simulink model "uav_simulation_tarot_r2022a"  (R2022a)
settings: Solver=ode45  StartTime=0.0  StopTime=sim_params.max_sim_time  FixedStep=uav.dynamics_srate  MaxStep=uav.dynamics_srate  MinStep=.001  RelTol=.01
undefined symbols (not defined in the file): deg, DiscIntNeverNeededParam, P_failure, processes, rad, s, sim_params, uav
libraries: aerolibconvert2 x2, shared6dof x1, dspstat3 x1
(part 1 of 2)
settings Model: Creator=Researcher  LastModifiedBy=oem
settings SolverCC: MaxConsecutiveMinStep=10  AlgebraicLoopSolver=TrustRegion
settings DataIOCC: ReturnWorkspaceOutputs=off
settings DebuggingCC: UnconnectedInputMsg=warning  UnconnectedOutputMsg=warning  UnconnectedLineMsg=warning  SFMachineParentedDataDiag=warning  ArithmeticOperatorsInVariantConditions=warning
settings SFSimCC: SimUseLocalCustomCode=off  CustomCodeUndefinedFunction=UseInterfaceOnly
settings RTWCC: RTWUseLocalCustomCode=off

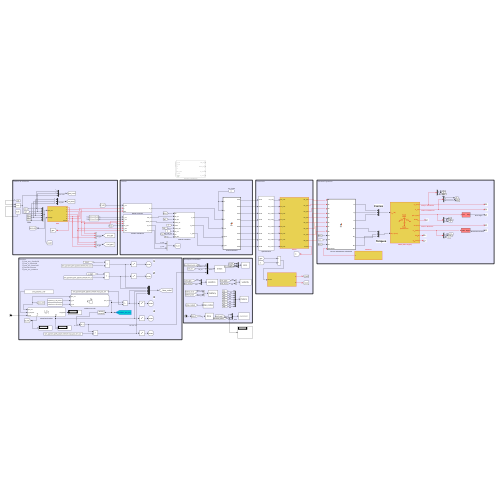
[thumbnail: Simulink's stored preview of the top-level diagram]
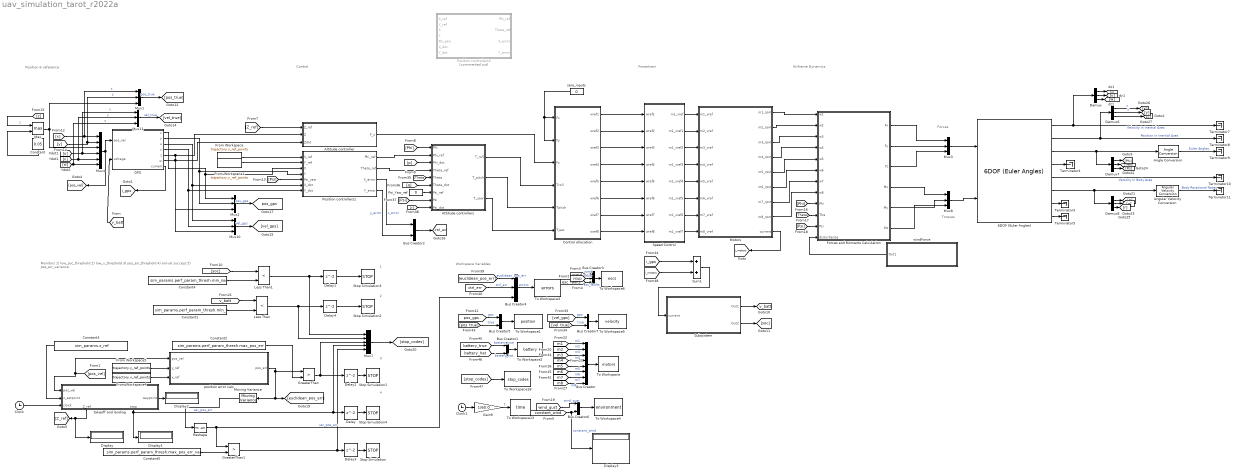
== system uav_simulation_tarot_r2022a ==
  note: Airframe Dynamics
  note: 1
  note: Monitors
      | 	1) low_soc_threshold
      | 	2) low_v_threshold
      | 	3) pos_err_threshold
      | 	4) arrival success
      |       5) pos_err_variance
  note: Powertrain
  note: Control
  note: 2
  note: 3
  note: 4
  note: Position & reference
  note: Workspace Variables
  note: Torques
  note: Forces
  6DOF (Euler Angles) : shared6dof/6DOF (Euler Angles)  units=Metric (MKS)  mtype=Fixed  rep=Quaternion  xme_0=[sim_params.initial_conditions.X, sim_params.initial_conditions.Y, sim_params.initial_conditions.Z]  Vm_0=[0 0 0]  eul_0=[0 0 0]  pm_0=[0 0 0]  mass_0=uav.mass  mass_e=0.5  mass_f=2.0  inertia=uav.airframe.Jb  inertia_e=eye(3)  inertia_f=2*eye(3)  k_quat=1.0  vre_flag=on  abi_flag=off  aMode=0  xme_statename=''  Vm_statename=''  eul_statename=''  quat_statename=''  pm_statename=''  mass_statename=''
      settings: SourceProductBaseCode=AE,PW,DR,MT,VE
  Altitude controller : Subsystem
  Angle Conversion : aerolibconvert2/Angle Conversion  IU=rad  OU=deg
  Angular Velocity Conversion : aerolibconvert2/Angular Velocity Conversion  IU=rad/s  OU=deg/s
  Attitude controllers : Subsystem
  Bus Creator : BusCreator  Inputs=8
  Bus Creator{1..2,5..7} (5 alike) : BusCreator  Inputs=2
  Bus Creator3 : BusCreator  Inputs=3
  Bus Creator4 : BusCreator  Inputs=3
  Clock : Clock
  Clock1 : Clock
  Constant : Constant  Value=0.05
  Constant1 : Constant  Value=sim_params.perf_param_thresh.min_v
  Constant2 : Constant  Value=sim_params.perf_param_thresh.max_pos_err
  Constant3 : Constant  Value=sim_params.z_ref
  Constant4 : Constant  Value=sim_params.perf_param_thresh.min_soc
  Constant5 : Constant  Value=sim_params.perf_param_thresh.max_pos_err_var
  Control allocation : MATLAB Function  TreatAsAtomicUnit=on
  Delay{,1..4} (5 alike) : Delay
  Demux{,6..8} (4 alike) : Demux  Outputs=3
  Display{,1..3} (4 alike) : Display
  Forces and Moments Calculation : MATLAB Function  TreatAsAtomicUnit=on
  From Workspace : FromWorkspace  VariableName=trajectory.x_ref_points
  From Workspace1 : FromWorkspace  VariableName=trajectory.y_ref_points
  From Workspace4 : FromWorkspace  VariableName=trajectory.x_ref_points
  From Workspace5 : FromWorkspace  VariableName=trajectory.y_ref_points
  GPS : Subsystem
  Gain9 : Gain  Gain=1/60.0
  GreaterThan : RelationalOperator  Operator=>  OutDataTypeStr=boolean  RndMeth=Simplest  InputSameDT=off
  GreaterThan1 : RelationalOperator  Operator=>  OutDataTypeStr=boolean  RndMeth=Simplest  InputSameDT=off
  Less Than : RelationalOperator  Operator=<  OutDataTypeStr=boolean  RndMeth=Simplest  InputSameDT=off
  Less Than1 : RelationalOperator  Operator=<  OutDataTypeStr=boolean  RndMeth=Simplest  InputSameDT=off
  Max : MinMax  Function=max  Inputs=2
  Motors : Subsystem
  Moving Variance : dspstat3/Moving Variance  Method=Sliding window  ForgettingFactorPort=off  SpecifyWindowLength=on  WindowLength=250  ForgettingFactor=0.9  SimulateUsing=Code generation
      settings: SourceProductBaseCode=DS
  Mux{1..3,8,10..11} (6 alike) : Mux  Inputs=3
  Mux4 : Mux  Inputs=6
  Mux7 : Mux  Inputs=5
  Position controllers1 : Subsystem
  Position controllers2 : Subsystem  Commented=on
  Psi_Yaw_ref : Constant  Value=0
  Reshape : Reshape
  Speed Control : Subsystem
  Stop Simulation{,1..4} (5 alike) : Stop
  Subsystem : Subsystem
  Sum1 : Sum
  Terminator{3..5,7..11} (8 alike) : Terminator
  To Workspace : ToWorkspace  VariableName=motors  SaveFormat=Timeseries  SampleTime=-1
  To Workspace1 : ToWorkspace  VariableName=position  SaveFormat=Timeseries  SampleTime=-1
  To Workspace13 : ToWorkspace  VariableName=time  SaveFormat=Timeseries  SampleTime=-1
  To Workspace18 : ToWorkspace  VariableName=stop_codes  SaveFormat=Timeseries  SampleTime=-1
  To Workspace2 : ToWorkspace  VariableName=battery  SaveFormat=Timeseries  SampleTime=-1
  To Workspace3 : ToWorkspace  VariableName=errors  SaveFormat=Timeseries  SampleTime=-1
  To Workspace4 : ToWorkspace  VariableName=environment  SaveFormat=Timeseries  SampleTime=-1
  To Workspace5 : ToWorkspace  VariableName=velocity  SaveFormat=Timeseries  SampleTime=-1
  To Workspace6 : ToWorkspace  VariableName=escs  SaveFormat=Timeseries  SampleTime=-1
  position error calc : Stateflow chart  TreatAsAtomicUnit=on
      settings: PortSchema="{\"entries\":[{\"content\":{\"sides\":[{\"content\":{\"connectorIds\":[\"In1\",\"In3\",\"In2\"]},\"type\":\"ConnectorPlacement.EquallySpacedRectSide\",\"uuid\":\"15dd5aaf-db5f-4100-8d44-c6b196b99d7e\"},{\"content\":{\"connectorIds\":[\"Out1\"],\"side\":\"RIGHT\"},\"type\":\"ConnectorPlacement.EquallySpacedRectSide\",\"uuid\":\"60222e26-82e5-4320-be9d-a2c6fe091c2c\"},{\"content\":{\"connectorIds\":[],\"side\":\"TOP\"},\"type\":\"ConnectorPlacement.EquallySpacedRectSide\",\"uuid\":\"f68d0c6c-3e4f-4411-aa05-b15e83a97581\"},{\"content\":{\"connectorIds\":[],\"side\":\"BOTTOM\"},\"type\":\"ConnectorPlacement.EquallySpacedRectSide\",\"uuid\":\"4c051fdf-ae8c-4c56-a072-e71b38b23a79\"}]},\"type\":\"ConnectorPlacement.EquallySpacedConnector\",\"uuid\":\"476607e2-95ee-46d1-bde8-442c90884603\"}],\"packageUris\":[\"http://schema.mathworks.com/mf0/Connector/R2020b\"],\"version\":\"1.0\"}"
  takeoff and landing : Stateflow chart  TreatAsAtomicUnit=on
      settings: PortSchema="{\"entries\":[{\"content\":{\"sides\":[{\"content\":{\"connectorIds\":[\"In1\",\"In2\",\"In3\"]},\"type\":\"ConnectorPlacement.EquallySpacedRectSide\",\"uuid\":\"11e534f3-7296-40bf-aaf5-6b635a6123b7\"},{\"content\":{\"connectorIds\":[\"Out1\"],\"side\":\"RIGHT\"},\"type\":\"ConnectorPlacement.EquallySpacedRectSide\",\"uuid\":\"0c003671-8499-4bdc-80ec-6f06b7f1861b\"},{\"content\":{\"connectorIds\":[],\"side\":\"TOP\"},\"type\":\"ConnectorPlacement.EquallySpacedRectSide\",\"uuid\":\"dd8fb418-d1e6-4628-bf44-6fc4ef2cf7ad\"},{\"content\":{\"connectorIds\":[\"Out2\",\"Out3\"],\"side\":\"BOTTOM\"},\"type\":\"ConnectorPlacement.EquallySpacedRectSide\",\"uuid\":\"62eca2cb-761d-4ce3-a85c-b402bb41b07d\"}]},\"type\":\"ConnectorPlacement.EquallySpacedConnector\",\"uuid\":\"b3efa352-b8bc-43a3-a44e-514725c3dafc\"}],\"packageUris\":[\"http://schema.mathworks.com/mf0/Connector/R2020b\"],\"version\":\"1.0\"}"
  windForce : Subsystem
  zero_inputs : Constant  Value=0
  tag scope: ctrl_err=global, i_gps=global, i_motors=global, pos_gps=global, v_batt=global
  wires:
  [y] -> Mux4/2, Mux1/2  "y"
  [x] -> Mux1/1, Mux4/1  "x"
  Attitude controllers/1(T_roll) -> Control allocation/4(Troll)
  Position controllers1/1(Phi_ref) -> Attitude controllers/2(Phi_ref)
  [r] -> Attitude controllers/9(Psi_dot)
  Attitude controllers/3(T_yaw) -> Control allocation/6(Tyaw)
  Bus Creator2/1 -> [ctrl_err]
  [Psi] -> Position controllers1/5(Psi_yaw)
  Position controllers1/3(X_error) -> Bus Creator2/1  "x_error"
  Attitude controllers/2(T_pitch) -> Control allocation/5(Tpitch)
  [Theta] -> Attitude controllers/5(Theta)
  Position controllers1/2(Theta_ref) -> Attitude controllers/4(Theta_ref)
  Altitude controller/1(F_z) -> Control allocation/3(Fz)
  [Phi] -> Attitude controllers/1(Phi)
  Position controllers1/4(Y_error) -> Bus Creator2/2  "y_error"
  [Psi] -> Attitude controllers/8(Psi)
  zero_inputs/1 -> Control allocation/1(Fx), Control allocation/2(Fy)
  [q] -> Attitude controllers/6(Theta_dot)
  Psi_Yaw_ref/1 -> Attitude controllers/7(Psi_ref)
  [p] -> Attitude controllers/3(Phi_dot)
  Mux7/1 -> [stop_codes]
  Gain9/1 -> To Workspace13/1  "t"
  Delay1/1 -> Stop Simulation3/1
  Constant4/1 -> Less Than1/2
  Clock1/1 -> Gain9/1
  [soc] -> Less Than1/1
  Less Than1/1 -> Delay1/1, Mux7/1
  [stop_codes] -> To Workspace18/1
  [pos_gps] -> Bus Creator5/1  "gps"
  [battery_true] -> Bus Creator1/1  "battery_true"
  [battery_hat] -> Bus Creator1/2  "battery_hat"
  Motors/9(current) -> [i_motors]
  Subsystem/1(Out1) -> [v_batt]
  Subsystem/2(Out2) -> [soc]
  windForce/1(Out1) -> Forces and Moments Calculation/12(disturbance)
  [m2] -> Bus Creator/2  "m2"
  Mux1/1 -> [pos_true]  "pos_true"
  Constant1/1 -> Less Than/2
  [v_batt] -> Less Than/1
  Delay4/1 -> Stop Simulation2/1
  Less Than/1 -> Mux7/2, Delay4/1
  [m1] -> Bus Creator/1  "m1"
  Bus Creator/1 -> To Workspace/1
  [m3] -> Bus Creator/3  "m3"
  [m4] -> Bus Creator/4  "m4"
  [m5] -> Bus Creator/5  "m5"
  [m6] -> Bus Creator/6  "m6"
  [m7] -> Bus Creator/7  "m7"
  [m8] -> Bus Creator/8  "m8"
  [pos_true] -> Bus Creator5/2  "true"
  Mux2/1 -> [pos_gps]  "pos_gps"
  Bus Creator1/1 -> To Workspace2/1
  [euclidean_pos_err] -> Bus Creator4/1  "euclidean_pos_err"
  [ctrl_err] -> Bus Creator4/2  "ctrl_err"
  Bus Creator4/1 -> To Workspace3/1  "errors"
  Bus Creator5/1 -> To Workspace1/1
  [wind_gust] -> Bus Creator6/1  "wind_gust"
  Bus Creator6/1 -> To Workspace4/1
  Forces and Moments Calculation/3(Fz) -> Mux3/3
  Forces and Moments Calculation/6(Mz) -> Mux8/3
  Angle Conversion/1 -> Terminator9/1  "Euler Angles"
  Mux3/1 -> 6DOF (Euler Angles)/1
  Forces and Moments Calculation/5(My) -> Mux8/2
  Angular Velocity Conversion/1 -> Terminator11/1  "Body Rotational Rates"
  Forces and Moments Calculation/2(Fy) -> Mux3/2
  Demux6/2 -> [y]  "y"
  Mux8/1 -> 6DOF (Euler Angles)/2
  6DOF (Euler Angles)/2 -> Terminator8/1, Demux6/1  "Position in Inertial Axes"
  Demux8/1 -> [p]
  Demux/3 -> [w]
  6DOF (Euler Angles)/8 -> Terminator5/1
  Demux6/1 -> [x]  "x"
  Demux7/2 -> [Theta]
  Forces and Moments Calculation/4(Mx) -> Mux8/1
  6DOF (Euler Angles)/7 -> Terminator3/1
  6DOF (Euler Angles)/6 -> Demux8/1, Angular Velocity Conversion/1
  Demux8/3 -> [r]
  Demux7/1 -> [Phi]
  Demux8/2 -> [q]
  6DOF (Euler Angles)/3 -> Demux7/1, Angle Conversion/1
  6DOF (Euler Angles)/4 -> Terminator4/1
  6DOF (Euler Angles)/1 -> Terminator7/1, Demux/1  "Velocity in Inertial Axes"
  Demux6/3 -> [z]
  Forces and Moments Calculation/1(Fx) -> Mux3/1
  6DOF (Euler Angles)/5 -> Terminator10/1  "Velocity in Body Axes"
  Demux7/3 -> [Psi]
  Demux/2 -> [v]
  Demux/1 -> [u]
  Motors/1(m1_rpm) -> Forces and Moments Calculation/1(w1)
  Motors/2(m2_rpm) -> Forces and Moments Calculation/2(w2)
  Motors/3(m3_rpm) -> Forces and Moments Calculation/3(w3)
  Motors/4(m4_rpm) -> Forces and Moments Calculation/4(w4)
  Motors/5(m5_rpm) -> Forces and Moments Calculation/5(w5)
  Motors/6(m6_rpm) -> Forces and Moments Calculation/6(w6)
  Motors/7(m7_rpm) -> Forces and Moments Calculation/7(w7)
  Motors/8(m8_rpm) -> Forces and Moments Calculation/8(w8)
  [Psi] -> Forces and Moments Calculation/11(Psi)
  [Theta] -> Forces and Moments Calculation/10(The)
  [Phi] -> Forces and Moments Calculation/9(Phi)
  [vel_gps] -> Bus Creator7/1  "gps"
  [vel_true] -> Bus Creator7/2  "true"
  Bus Creator7/1 -> To Workspace5/1
  [v] -> Mux11/2, Mux4/5  "y"
  Mux10/1 -> [vel_gps]  "vel_gps"
  [w] -> Mux11/3, Mux4/6  "z"
  [u] -> Mux11/1, Mux4/4  "x"
  Mux11/1 -> [vel_true]  "vel_true"
  GPS/3(u) -> Mux10/1, Position controllers1/6(X_dot)
  GPS/4(v) -> Mux10/2, Position controllers1/7(Y_dot)
  GPS/2(y) -> Mux2/2, Position controllers1/4(Y)
  GPS/1(x) -> Position controllers1/3(X), Mux2/1
  Mux4/1 -> [pos_vel], GPS/1(pos_vel)
  GPS/5(z) -> Mux2/3, Altitude controller/2(Z)
  GPS/6(w) -> Mux10/3, Altitude controller/3(Zdot)
  [v_batt] -> GPS/2(voltage)
  GPS/7(current) -> [i_gps]
  Sum1/1 -> Subsystem/1(current)
  [i_gps] -> Sum1/1
  [i_motors] -> Sum1/2
  Constant/1 -> Max/2
  [z] -> Max/1  "z"
  Max/1 -> Mux4/3, Mux1/3
  Delay/1 -> Stop Simulation4/1
  [pos_vel] -> position error calc/1(pos_vel), takeoff and landing/1(pos_vel)
  takeoff and landing/2(Z_ref) -> Display/1, [Z_ref]
  [Z_ref] -> Altitude controller/1(Z_ref)
  From Workspace5/1 -> position error calc/3(y_ref)
  From Workspace4/1 -> position error calc/2(x_ref)
  Constant2/1 -> GreaterThan/2
  Delay2/1 -> Stop Simulation1/1
  GreaterThan/1 -> Mux7/3, Delay2/1
  takeoff and landing/3(stop) -> Mux7/4, Delay/1, Display1/1
  Control allocation/1(wref1) -> Speed Control/1(wref1)
  Control allocation/2(wref2) -> Speed Control/2(wref2)
  Control allocation/3(wref3) -> Speed Control/3(wref3)
  Control allocation/4(wref4) -> Speed Control/4(wref4)
  Control allocation/5(wref5) -> Speed Control/5(wref5)
  Control allocation/6(wref6) -> Speed Control/6(wref6)
  Control allocation/7(wref7) -> Speed Control/7(wref7)
  Control allocation/8(wref8) -> Speed Control/8(wref8)
  Speed Control/1(m1_vref) -> Motors/1(m1_vref)
  Speed Control/2(m1_vref1) -> Motors/2(m2_vref)
  Speed Control/3(m1_vref2) -> Motors/3(m3_vref)
  Speed Control/4(m1_vref3) -> Motors/4(m4_vref)
  Speed Control/5(m1_vref4) -> Motors/5(m5_vref)
  Speed Control/6(m1_vref5) -> Motors/6(m6_vref)
  Speed Control/7(m1_vref6) -> Motors/7(m7_vref)
  Speed Control/8(m1_vref7) -> Motors/8(m8_vref)
  Constant3/1 -> takeoff and landing/2(z_setpoint)
  Clock/1 -> takeoff and landing/3(clock)
  From Workspace/1 -> Position controllers1/1(X_ref)
  From Workspace1/1 -> Position controllers1/2(Y_ref)
  [esc_faults] -> Bus Creator3/3  "esc_faults"
  Bus Creator3/1 -> To Workspace6/1
  [vcmd] -> Bus Creator3/1  "vcmd"
  [vsup] -> Bus Creator3/2  "vsup"
  position error calc/1(pos_err) -> GreaterThan/1, [euclidean_pos_err], Moving Variance/1
  Moving Variance/1 -> Reshape/1  "var_pos_err"
  Reshape/1 -> GreaterThan1/1, Bus Creator4/3  "var_pos_err"
  Constant5/1 -> GreaterThan1/2
  GreaterThan1/1 -> Mux7/5, Delay3/1
  takeoff and landing/1(waypoint) -> Display2/1
  Delay3/1 -> Stop Simulation/1
  [constant_wind] -> Display3/1, Bus Creator6/2  "constant_wind"

== system uav_simulation_tarot_r2022a/Altitude controller ==
  Z_ref : Inport
  Z : Inport  Port=2
  Zdot : Inport  Port=3
  Add : Sum  Inputs=+++
  Add2 : Sum  Inputs=+-
  Constant2 : Constant  Value=9.8*uav.mass
  Kdz : Gain  Gain=-6.0
  Kpz : Gain  Gain=-6.0
  mass : Gain  Gain=uav.mass
  mass1 : Gain  Gain=uav.mass
  F_z : Outport  VectorParamsAs1DForOutWhenUnconnected=off
  wires:
  Add2/1 -> Kpz/1
  Constant2/1 -> Add/1
  Z/1 -> Add2/1
  Z_ref/1 -> Add2/2
  Zdot/1 -> Kdz/1
  Kpz/1 -> mass/1
  Kdz/1 -> mass1/1
  mass1/1 -> Add/3
  mass/1 -> Add/2
  Add/1 -> F_z/1

== system uav_simulation_tarot_r2022a/Attitude controllers ==
  Phi : Inport
  Phi_ref : Inport  Port=2
  Phi_dot : Inport  Port=3
  Theta_ref : Inport  Port=4
  Theta : Inport  Port=5
  Theta_dot : Inport  Port=6
  Psi_ref : Inport  Port=7
  Psi : Inport  Port=8
  Psi_dot : Inport  Port=9
  PD_pitch : Subsystem
  PD_roll : Subsystem
  PD_yaw : Subsystem
  T_roll : Outport  VectorParamsAs1DForOutWhenUnconnected=off
  T_pitch : Outport  Port=2  VectorParamsAs1DForOutWhenUnconnected=off
  T_yaw : Outport  Port=3  VectorParamsAs1DForOutWhenUnconnected=off
  wires:
  PD_yaw/1(Tyaw) -> T_yaw/1
  PD_roll/1(Troll) -> T_roll/1
  Theta_ref/1 -> PD_pitch/1(Theta_ref)
  Theta_dot/1 -> PD_pitch/3(Theta_dot)
  PD_pitch/1(Tpitch) -> T_pitch/1
  Phi/1 -> PD_roll/2(Phi)
  Psi_dot/1 -> PD_yaw/3(Psi_dot)
  Psi_ref/1 -> PD_yaw/1(Psi_ref)
  Theta/1 -> PD_pitch/2(Theta)
  Phi_dot/1 -> PD_roll/3(Phi_dot)
  Psi/1 -> PD_yaw/2(Psi)
  Phi_ref/1 -> PD_roll/1(Phi_ref)

== system uav_simulation_tarot_r2022a/GPS ==
  pos_vel : Inport
  voltage : Inport  Port=2
  Clock : Clock
  Demux1 : Demux  Outputs=6
  Divide : Product  Inputs=*/
  GPS_Vs : Saturate  UpperLimit=uav.gps.voltage_supply  LowerLimit=uav.gps.voltage_supply
  GPS_Watts : RandomNumber  Mean=double(uav.gps.avg_watts)  Variance=double(uav.gps.std_watts)  SampleTime=1
  measurement : MATLAB Function  TreatAsAtomicUnit=on  SystemSampleTime=uav.dynamics_srate
  x : Outport
  y : Outport  Port=2
  u : Outport  Port=3
  v : Outport  Port=4
  z : Outport  Port=5
  w : Outport  Port=6
  current : Outport  Port=7
  wires:
  Demux1/4 -> u/1  "u"
  Demux1/2 -> y/1  "y"
  Demux1/5 -> v/1  "v"
  Clock/1 -> measurement/2(t)
  pos_vel/1 -> measurement/1(u)
  measurement/1(y) -> Demux1/1
  Demux1/6 -> w/1  "w"
  Demux1/3 -> z/1  "z"
  Demux1/1 -> x/1  "x"
  voltage/1 -> GPS_Vs/1
  GPS_Watts/1 -> Divide/1
  GPS_Vs/1 -> Divide/2
  Divide/1 -> current/1

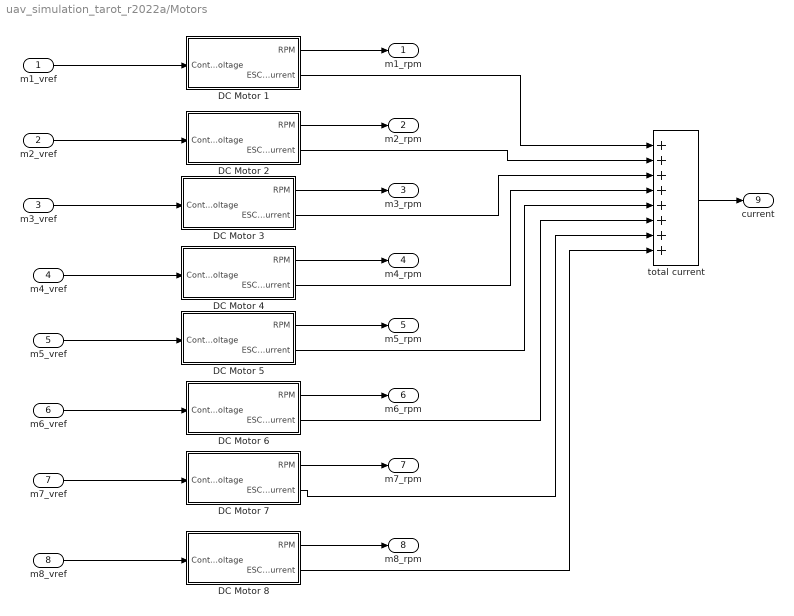
== system uav_simulation_tarot_r2022a/Motors ==
  m1_vref : Inport
  m2_vref : Inport  Port=2
  m3_vref : Inport  Port=3
  m4_vref : Inport  Port=4
  m5_vref : Inport  Port=5
  m6_vref : Inport  Port=6
  m7_vref : Inport  Port=7
  m8_vref : Inport  Port=8
  DC Motor 1 : Subsystem
  DC Motor 2 : Subsystem
  DC Motor 3 : Subsystem
  DC Motor 4 : Subsystem
  DC Motor 5 : Subsystem
  DC Motor 6 : Subsystem
  DC Motor 7 : Subsystem
  DC Motor 8 : Subsystem
  total current : Sum  Inputs=++++++++
  m1_rpm : Outport  VectorParamsAs1DForOutWhenUnconnected=off
  m2_rpm : Outport  Port=2  VectorParamsAs1DForOutWhenUnconnected=off
  m3_rpm : Outport  Port=3  VectorParamsAs1DForOutWhenUnconnected=off
  m4_rpm : Outport  Port=4  VectorParamsAs1DForOutWhenUnconnected=off
  m5_rpm : Outport  Port=5  VectorParamsAs1DForOutWhenUnconnected=off
  m6_rpm : Outport  Port=6  VectorParamsAs1DForOutWhenUnconnected=off
  m7_rpm : Outport  Port=7  VectorParamsAs1DForOutWhenUnconnected=off
  m8_rpm : Outport  Port=8  VectorParamsAs1DForOutWhenUnconnected=off
  current : Outport  Port=9  VectorParamsAs1DForOutWhenUnconnected=off
  wires:
  DC Motor 6/2(ESC Current) -> total current/6
  DC Motor 7/2(ESC Current) -> total current/7
  DC Motor 5/2(ESC Current) -> total current/5
  DC Motor 8/2(ESC Current) -> total current/8
  DC Motor 1/2(ESC Current) -> total current/1
  DC Motor 2/2(ESC Current) -> total current/2
  DC Motor 4/2(ESC Current) -> total current/4
  DC Motor 3/2(ESC Current) -> total current/3
  DC Motor 5/1(RPM) -> m5_rpm/1
  DC Motor 7/1(RPM) -> m7_rpm/1
  DC Motor 2/1(RPM) -> m2_rpm/1
  DC Motor 3/1(RPM) -> m3_rpm/1
  DC Motor 4/1(RPM) -> m4_rpm/1
  DC Motor 6/1(RPM) -> m6_rpm/1
  DC Motor 8/1(RPM) -> m8_rpm/1
  DC Motor 1/1(RPM) -> m1_rpm/1
  m7_vref/1 -> DC Motor 7/1(Control  Voltage)
  m8_vref/1 -> DC Motor 8/1(Control  Voltage)
  m6_vref/1 -> DC Motor 6/1(Control  Voltage)
  m5_vref/1 -> DC Motor 5/1(Control  Voltage)
  m4_vref/1 -> DC Motor 4/1(Control  Voltage)
  m3_vref/1 -> DC Motor 3/1(Control  Voltage)
  m2_vref/1 -> DC Motor 2/1(Control  Voltage)
  total current/1 -> current/1
  m1_vref/1 -> DC Motor 1/1(Control  Voltage)

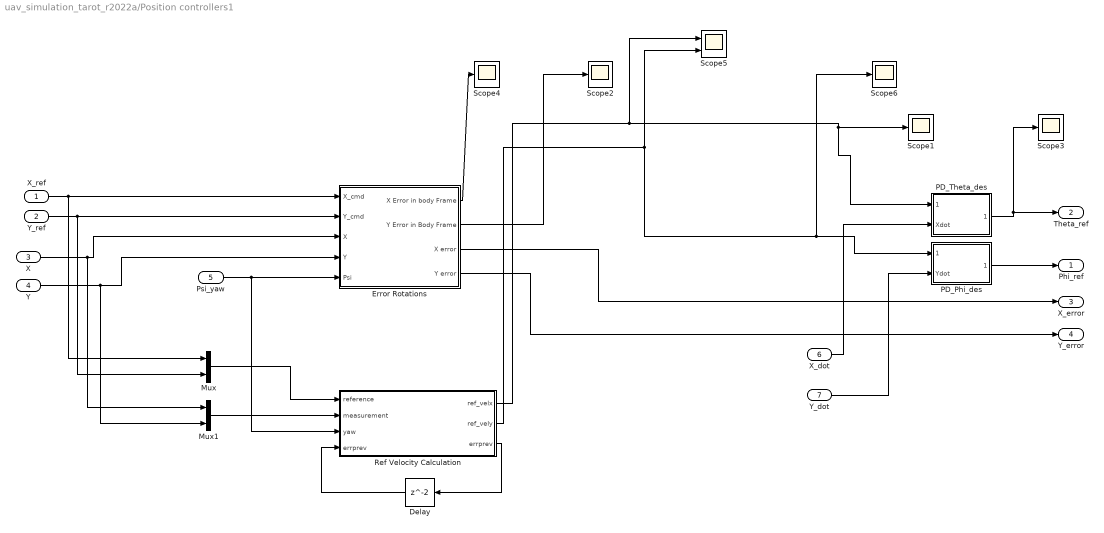
== system uav_simulation_tarot_r2022a/Position controllers1 ==
  X_ref : Inport
  Y_ref : Inport  Port=2
  X : Inport  Port=3
  Y : Inport  Port=4
  Psi_yaw : Inport  Port=5
  X_dot : Inport  Port=6
  Y_dot : Inport  Port=7
  Delay : Delay  SampleTime=uav.dynamics_srate
  Error Rotations : Subsystem
  Mux : Mux  Inputs=2
  Mux1 : Mux  Inputs=2
  PD_Phi_des : Subsystem
  PD_Theta_des : Subsystem
  Ref Velocity Calculation : MATLAB Function  TreatAsAtomicUnit=on
  Scope{1..4,6} (5 alike) : Scope
  Scope5 : Scope  NumInputPorts=2
  Phi_ref : Outport  VectorParamsAs1DForOutWhenUnconnected=off
  Theta_ref : Outport  Port=2  VectorParamsAs1DForOutWhenUnconnected=off
  X_error : Outport  Port=3  VectorParamsAs1DForOutWhenUnconnected=off
  Y_error : Outport  Port=4  VectorParamsAs1DForOutWhenUnconnected=off
  wires:
  X/1 -> Mux1/1, Error Rotations/3(X)
  PD_Phi_des/1(Phi_des) -> Phi_ref/1
  Ref Velocity Calculation/2(ref_vely) -> Scope6/1, PD_Phi_des/1(Ydot_ref), Scope5/2
  X_dot/1 -> PD_Theta_des/2(Xdot)
  PD_Theta_des/1(Theta_des) -> Scope3/1, Theta_ref/1
  Psi_yaw/1 -> Ref Velocity Calculation/3(yaw), Error Rotations/5(Psi)
  Y_ref/1 -> Mux/2, Error Rotations/2(Y_cmd)
  Error Rotations/4("Y error ") -> Y_error/1
  Y_dot/1 -> PD_Phi_des/2(Ydot)
  Error Rotations/3(X error) -> X_error/1
  X_ref/1 -> Mux/1, Error Rotations/1(X_cmd)
  Ref Velocity Calculation/1(ref_velx) -> PD_Theta_des/1(Xdot_ref), Scope1/1, Scope5/1
  Y/1 -> Mux1/2, Error Rotations/4(Y)
  Mux/1 -> Ref Velocity Calculation/1(reference)
  Mux1/1 -> Ref Velocity Calculation/2(measurement)
  Ref Velocity Calculation/3(errprev) -> Delay/1
  Delay/1 -> Ref Velocity Calculation/4("errprev ")
  Error Rotations/1(X Error in body Frame) -> Scope4/1
  Error Rotations/2(Y Error in Body Frame) -> Scope2/1

== system uav_simulation_tarot_r2022a/Position controllers2 ==
  X_ref : Inport
  Y_ref : Inport  Port=2
  X : Inport  Port=3
  Y : Inport  Port=4
  Psi_yaw : Inport  Port=5
  X_dot : Inport  Port=6
  Y_dot : Inport  Port=7
  Error Rotations : Subsystem
  PD_Phi_des : Subsystem
  PD_Theta_des : Subsystem
  Phi_ref : Outport  VectorParamsAs1DForOutWhenUnconnected=off
  Theta_ref : Outport  Port=2  VectorParamsAs1DForOutWhenUnconnected=off
  X_error : Outport  Port=3  VectorParamsAs1DForOutWhenUnconnected=off
  Y_error : Outport  Port=4  VectorParamsAs1DForOutWhenUnconnected=off
  wires:
  Y/1 -> Error Rotations/4(Y)
  Y_ref/1 -> Error Rotations/2(Y_cmd)
  Error Rotations/4("Y error ") -> Y_error/1
  Error Rotations/3(X error) -> X_error/1
  Error Rotations/1(X Error in body Frame) -> PD_Theta_des/1(Xdot_ref)
  X/1 -> Error Rotations/3(X)
  Y_dot/1 -> PD_Phi_des/2(Ydot)
  PD_Phi_des/1(Phi_des) -> Phi_ref/1
  Error Rotations/2(Y Error in Body Frame) -> PD_Phi_des/1(Ydot_ref)
  Psi_yaw/1 -> Error Rotations/5(Psi)
  PD_Theta_des/1(Theta_des) -> Theta_ref/1
  X_dot/1 -> PD_Theta_des/2(Xdot)
  X_ref/1 -> Error Rotations/1(X_cmd)

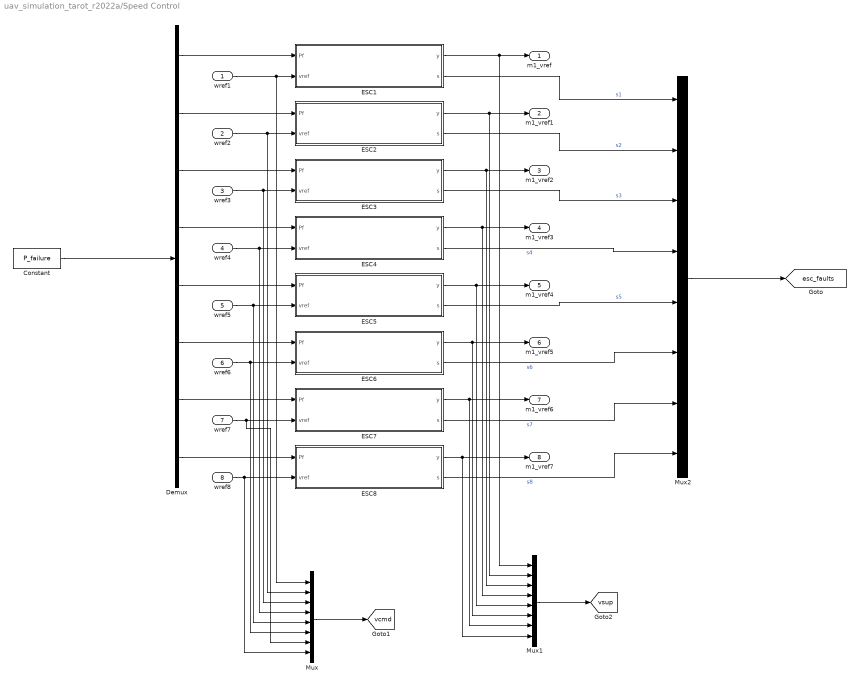
== system uav_simulation_tarot_r2022a/Speed Control ==
  wref1 : Inport
  wref2 : Inport  Port=2
  wref3 : Inport  Port=3
  wref4 : Inport  Port=4
  wref5 : Inport  Port=5
  wref6 : Inport  Port=6
  wref7 : Inport  Port=7
  wref8 : Inport  Port=8
  Constant : Constant  Value=P_failure
  Demux : Demux  Outputs=length(uav.motors)
  ESC1 : Subsystem
  ESC2 : Subsystem
  ESC3 : Subsystem
  ESC4 : Subsystem
  ESC5 : Subsystem
  ESC6 : Subsystem
  ESC7 : Subsystem
  ESC8 : Subsystem
  Mux : Mux  Inputs=8
  Mux1 : Mux  Inputs=8
  Mux2 : Mux  Inputs=8
  m1_vref : Outport
  m1_vref1 : Outport  Port=2
  m1_vref2 : Outport  Port=3
  m1_vref3 : Outport  Port=4
  m1_vref4 : Outport  Port=5
  m1_vref5 : Outport  Port=6
  m1_vref6 : Outport  Port=7
  m1_vref7 : Outport  Port=8
  tag scope: esc_faults=global, vcmd=global, vsup=global
  wires:
  Constant/1 -> Demux/1
  Demux/1 -> ESC1/1(Pf)
  wref1/1 -> Mux/1, ESC1/2(vref)
  wref2/1 -> Mux/2, ESC2/2(vref)
  Demux/2 -> ESC2/1(Pf)
  Demux/3 -> ESC3/1(Pf)
  wref3/1 -> Mux/3, ESC3/2(vref)
  Demux/4 -> ESC4/1(Pf)
  wref4/1 -> Mux/4, ESC4/2(vref)
  Demux/5 -> ESC5/1(Pf)
  wref5/1 -> Mux/5, ESC5/2(vref)
  Demux/6 -> ESC6/1(Pf)
  wref6/1 -> Mux/6, ESC6/2(vref)
  Demux/7 -> ESC7/1(Pf)
  wref7/1 -> Mux/7, ESC7/2(vref)
  Demux/8 -> ESC8/1(Pf)
  wref8/1 -> Mux/8, ESC8/2(vref)
  ESC4/2(s) -> Mux2/4  "s4"
  ESC5/2(s) -> Mux2/5  "s5"
  ESC1/2(s) -> Mux2/1  "s1"
  ESC2/2(s) -> Mux2/2  "s2"
  ESC3/2(s) -> Mux2/3  "s3"
  ESC6/2(s) -> Mux2/6  "s6"
  ESC7/2(s) -> Mux2/7  "s7"
  ESC8/2(s) -> Mux2/8  "s8"
  Mux2/1 -> [esc_faults]
  Mux/1 -> [vcmd]
  ESC7/1(y) -> m1_vref6/1, Mux1/7
  ESC6/1(y) -> Mux1/6, m1_vref5/1
  ESC2/1(y) -> Mux1/2, m1_vref1/1
  ESC8/1(y) -> Mux1/8, m1_vref7/1
  ESC4/1(y) -> Mux1/4, m1_vref3/1
  ESC5/1(y) -> Mux1/5, m1_vref4/1
  ESC3/1(y) -> Mux1/3, m1_vref2/1
  Mux1/1 -> [vsup]
  ESC1/1(y) -> Mux1/1, m1_vref/1

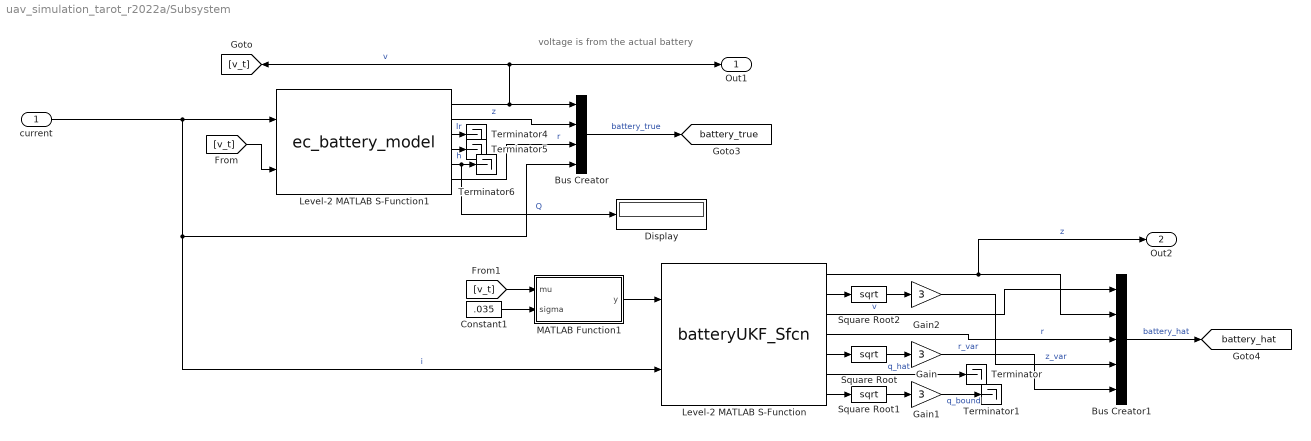
== system uav_simulation_tarot_r2022a/Subsystem ==
  note: voltage is from the actual battery
  current : Inport
  Bus Creator : BusCreator  Inputs=4
  Bus Creator1 : BusCreator  Inputs=5
  Constant1 : Constant  Value=.035
  Display : Display
  Gain : Gain  Gain=3
  Gain1 : Gain  Gain=3
  Gain2 : Gain  Gain=3
  Level-2 MATLAB S-Function : M-S-Function  FunctionName=batteryUKF_Sfcn  Parameters=uav.battery, uav.battery.dt, sim_params.battery_estimator
      mask Display:
      | port_label('input', 1, 'voltage');
      | port_label('input', 2, 'current');
      | port_label('output', 1, 'soc_hat');
      | port_label('output', 2, 'soc_bound');
      | port_label('output', 3, 'voltage_hat');
      | port_label('output', 4, 'r0_hat');
      | port_label('output', 5, 'r0_bound');
      | port_label('output', 6, 'q_hat');
      | port_label('output', 7, 'q_bound');
      | 
      | disp("UKF");
  Level-2 MATLAB S-Function1 : M-S-Function  FunctionName=ec_battery_model  Parameters=uav.battery
      mask Display:
      | port_label('output', 1, 'v');
      | port_label('output', 2, 'z');
      | port_label('output', 3, 'Ir');
      | port_label('output', 4, 'h');
      | port_label('output', 5, 'Q');
      | port_label('output', 6, 'R0');
      | 
      | port_label('input', 1, 'u');
      | port_label('input', 2, 'v_(t-1)');
  MATLAB Function1 : MATLAB Function  TreatAsAtomicUnit=on
  Square Root : Sqrt
  Square Root1 : Sqrt
  Square Root2 : Sqrt
  Terminator{,1,4..6} (5 alike) : Terminator
  Out1 : Outport
  Out2 : Outport  Port=2
  tag scope: battery_hat=global, battery_true=global
  wires:
  MATLAB Function1/1(y) -> Level-2 MATLAB S-Function/1
  Constant1/1 -> MATLAB Function1/2(sigma)
  Level-2 MATLAB S-Function/5 -> Square Root/1
  Square Root/1 -> Gain/1
  Bus Creator/1 -> [battery_true]  "battery_true"
  Square Root1/1 -> Gain1/1
  Square Root2/1 -> Gain2/1
  Level-2 MATLAB S-Function/2 -> Square Root2/1
  Level-2 MATLAB S-Function/7 -> Square Root1/1
  Level-2 MATLAB S-Function/3 -> Bus Creator1/1  "v"
  Level-2 MATLAB S-Function/1 -> Out2/1, Bus Creator1/2  "z"
  Gain2/1 -> Bus Creator1/4  "z_var"
  Level-2 MATLAB S-Function/4 -> Bus Creator1/3  "r"
  Gain/1 -> Bus Creator1/5  "r_var"
  Gain1/1 -> Terminator1/1  "q_bound"
  Bus Creator1/1 -> [battery_hat]  "battery_hat"
  current/1 -> Level-2 MATLAB S-Function/2, Bus Creator/4, Level-2 MATLAB S-Function1/1  "i"
  Level-2 MATLAB S-Function/6 -> Terminator/1  "q_hat"
  Level-2 MATLAB S-Function1/3 -> Terminator4/1  "Ir"
  Level-2 MATLAB S-Function1/4 -> Terminator5/1  "h"
  Level-2 MATLAB S-Function1/5 -> Display/1, Terminator6/1  "Q"
  [v_t] -> Level-2 MATLAB S-Function1/2
  Level-2 MATLAB S-Function1/1 -> Out1/1, [v_t], Bus Creator/1  "v"
  Level-2 MATLAB S-Function1/2 -> Bus Creator/2  "z"
  Level-2 MATLAB S-Function1/6 -> Bus Creator/3  "r"
  [v_t] -> MATLAB Function1/1(mu)

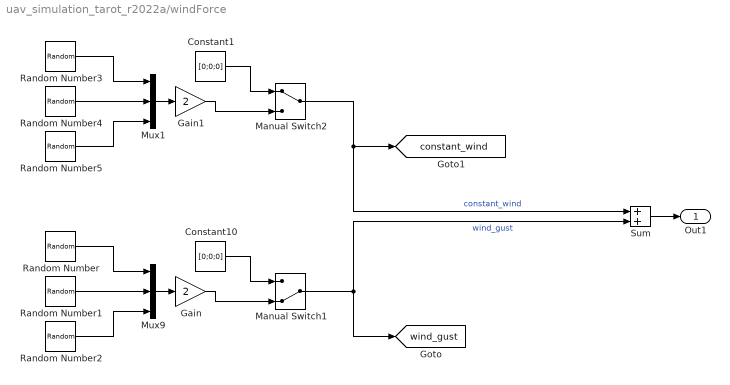
== system uav_simulation_tarot_r2022a/windForce ==
  Constant1 : Constant  Value=[0;0;0]
  Constant10 : Constant  Value=[0;0;0]
  Gain : Gain  Gain=2
  Gain1 : Gain  Gain=2
  Manual Switch1 : ManualSwitch  CurrentSetting=0
  Manual Switch2 : ManualSwitch
  Mux1 : Mux  Inputs=3
  Mux9 : Mux  Inputs=3
  Random Number : RandomNumber  Mean=processes.environment.wind.gust.x(1)  Variance=processes.environment.wind.gust.x(2)  Seed=round(rand*1000000)  SampleTime=1
  Random Number1 : RandomNumber  Mean=processes.environment.wind.gust.y(1)  Variance=processes.environment.wind.gust.y(2)  Seed=round(rand*1000000)  SampleTime=1
  Random Number2 : RandomNumber  Mean=processes.environment.wind.gust.z(1)  Variance=processes.environment.wind.gust.z(2)  Seed=round(rand*100000)  SampleTime=1
  Random Number3 : RandomNumber  Mean=2  Variance=1.5  Seed=round(rand*1000000)  SampleTime=50
  Random Number4 : RandomNumber  Mean=2  Variance=1.5  Seed=round(rand*1000000)  SampleTime=50
  Random Number5 : RandomNumber  Seed=round(rand*100000)  SampleTime=50
  Sum : Sum
  Out1 : Outport
  tag scope: constant_wind=global, wind_gust=global
  wires:
  Random Number1/1 -> Mux9/2
  Mux9/1 -> Gain/1
  Manual Switch1/1 -> Sum/2, [wind_gust]  "wind_gust"
  Random Number2/1 -> Mux9/3
  Random Number/1 -> Mux9/1
  Constant10/1 -> Manual Switch1/1
  Gain/1 -> Manual Switch1/2
  Random Number4/1 -> Mux1/2
  Constant1/1 -> Manual Switch2/1
  Random Number5/1 -> Mux1/3
  Manual Switch2/1 -> Sum/1, [constant_wind]  "constant_wind"
  Gain1/1 -> Manual Switch2/2
  Random Number3/1 -> Mux1/1
  Mux1/1 -> Gain1/1
  Sum/1 -> Out1/1

== system uav_simulation_tarot_r2022a/Attitude controllers/PD_pitch ==
  Theta_ref : Inport
  Theta : Inport  Port=2
  Theta_dot : Inport  Port=3
  Add : Sum  Inputs=-+
  Gain : Gain  Gain=4
  Gain1 : Gain  Gain=1.25
  Gain2 : Gain  Gain=-1
  Sum : Sum  Inputs=|++
  Tpitch : Outport  VectorParamsAs1DForOutWhenUnconnected=off
  wires:
  Gain2/1 -> Tpitch/1
  Gain/1 -> Sum/1
  Theta/1 -> Add/2
  Add/1 -> Gain/1
  Gain1/1 -> Sum/2
  Sum/1 -> Gain2/1
  Theta_dot/1 -> Gain1/1
  Theta_ref/1 -> Add/1

== system uav_simulation_tarot_r2022a/Attitude controllers/PD_roll ==
  Phi_ref : Inport
  Phi : Inport  Port=2
  Phi_dot : Inport  Port=3
  Add : Sum  Inputs=-+
  Gain : Gain  Gain=3
  Gain1 : Gain
  Gain2 : Gain  Gain=-1
  Sum : Sum  Inputs=|++
  Troll : Outport  VectorParamsAs1DForOutWhenUnconnected=off
  wires:
  Phi_ref/1 -> Add/1
  Phi_dot/1 -> Gain1/1
  Sum/1 -> Gain2/1
  Gain1/1 -> Sum/2
  Add/1 -> Gain/1
  Phi/1 -> Add/2
  Gain/1 -> Sum/1
  Gain2/1 -> Troll/1

== system uav_simulation_tarot_r2022a/Attitude controllers/PD_yaw ==
  Psi_ref : Inport
  Psi : Inport  Port=2
  Psi_dot : Inport  Port=3
  Add : Sum  Inputs=-+
  Gain : Gain  Gain=3
  Gain1 : Gain
  Gain2 : Gain  Gain=-1
  Sum : Sum  Inputs=|++
  Tyaw : Outport  VectorParamsAs1DForOutWhenUnconnected=off
  wires:
  Psi_ref/1 -> Add/1
  Psi_dot/1 -> Gain1/1
  Sum/1 -> Gain2/1
  Gain1/1 -> Sum/2
  Add/1 -> Gain/1
  Psi/1 -> Add/2
  Gain/1 -> Sum/1
  Gain2/1 -> Tyaw/1

== system uav_simulation_tarot_r2022a/Motors/DC Motor 1 ==
  Control  Voltage : Inport
  Bus Creator : BusCreator  Inputs=4
  Electrical part : Subsystem
  Mechanical part : Subsystem
  Scope : Scope
  StaticTfric : Constant  Value=0
  RPM : Outport  VectorParamsAs1DForOutWhenUnconnected=off
  ESC Current : Outport  Port=2  VectorParamsAs1DForOutWhenUnconnected=off
  tag scope: m1=global
  wires:
  StaticTfric/1 -> Mechanical part/2(Static Friction Torque)
  Control  Voltage/1 -> Bus Creator/4, Electrical part/1(ESC voltage)  "vref"
  Bus Creator/1 -> [m1]  "m1"
  Mechanical part/1(rpm) -> RPM/1, Bus Creator/1  "rpm"
  Electrical part/1(Electrical Torque) -> Mechanical part/1(Electrical Torque)  "torque"
  Electrical part/2(current) -> ESC Current/1, Bus Creator/3  "current"
  Mechanical part/2(torque) -> Scope/1, Bus Creator/2  "torque"
  Mechanical part/3(angular_speed) -> Electrical part/2(w angular speed)

== system uav_simulation_tarot_r2022a/Motors/DC Motor 2 ==
  Control  Voltage : Inport
  Bus Creator : BusCreator  Inputs=4
  Electrical part : Subsystem
  Mechanical part : Subsystem
  StaticTfric : Constant  Value=0
  RPM : Outport  VectorParamsAs1DForOutWhenUnconnected=off
  ESC Current : Outport  Port=2  VectorParamsAs1DForOutWhenUnconnected=off
  tag scope: m2=global
  wires:
  StaticTfric/1 -> Mechanical part/2(Static Friction Torque)
  Control  Voltage/1 -> Bus Creator/4, Electrical part/1(ESC voltage)  "vref"
  Bus Creator/1 -> [m2]  "m2"
  Mechanical part/1(rpm) -> RPM/1, Bus Creator/1  "rpm"
  Electrical part/1(Electrical Torque) -> Mechanical part/1(Electrical Torque)  "torque"
  Electrical part/2(current) -> ESC Current/1, Bus Creator/3  "current"
  Mechanical part/2(torque) -> Bus Creator/2  "torque"
  Mechanical part/3(angular_velocity) -> Electrical part/2(w angular speed)

== system uav_simulation_tarot_r2022a/Motors/DC Motor 3 ==
  Control  Voltage : Inport
  Bus Creator : BusCreator  Inputs=4
  Electrical part : Subsystem
  Mechanical part : Subsystem
  StaticTfric : Constant  Value=0
  RPM : Outport  VectorParamsAs1DForOutWhenUnconnected=off
  ESC Current : Outport  Port=2  VectorParamsAs1DForOutWhenUnconnected=off
  tag scope: m3=global
  wires:
  StaticTfric/1 -> Mechanical part/2(Static Friction Torque)
  Control  Voltage/1 -> Bus Creator/4, Electrical part/1(ESC voltage)  "vref"
  Bus Creator/1 -> [m3]  "m3"
  Mechanical part/1(rpm) -> RPM/1, Bus Creator/1  "rpm"
  Electrical part/1(Electrical Torque) -> Mechanical part/1(Electrical Torque)  "torque"
  Electrical part/2(current) -> ESC Current/1, Bus Creator/3  "current"
  Mechanical part/2(torque) -> Bus Creator/2  "torque"
  Mechanical part/3(angular_velocity) -> Electrical part/2(w angular speed)

== system uav_simulation_tarot_r2022a/Motors/DC Motor 4 ==
  Control  Voltage : Inport
  Bus Creator : BusCreator  Inputs=4
  Electrical part : Subsystem
  Mechanical part : Subsystem
  StaticTfric : Constant  Value=0
  RPM : Outport  VectorParamsAs1DForOutWhenUnconnected=off
  ESC Current : Outport  Port=2  VectorParamsAs1DForOutWhenUnconnected=off
  tag scope: m4=global
  wires:
  StaticTfric/1 -> Mechanical part/2(Static Friction Torque)
  Control  Voltage/1 -> Bus Creator/4, Electrical part/1(ESC voltage)  "vref"
  Bus Creator/1 -> [m4]  "m4"
  Mechanical part/1(rpm) -> RPM/1, Bus Creator/1  "rpm"
  Electrical part/1(Electrical Torque) -> Mechanical part/1(Electrical Torque)  "torque"
  Electrical part/2(current) -> ESC Current/1, Bus Creator/3  "current"
  Mechanical part/2(torque) -> Bus Creator/2  "torque"
  Mechanical part/3(angular_velocity) -> Electrical part/2(w angular speed)

== system uav_simulation_tarot_r2022a/Motors/DC Motor 5 ==
  Control  Voltage : Inport
  Bus Creator : BusCreator  Inputs=4
  Electrical part : Subsystem
  Mechanical part : Subsystem
  StaticTfric : Constant  Value=0
  RPM : Outport  VectorParamsAs1DForOutWhenUnconnected=off
  ESC Current : Outport  Port=2  VectorParamsAs1DForOutWhenUnconnected=off
  tag scope: m5=global
  wires:
  StaticTfric/1 -> Mechanical part/2(Static Friction Torque)
  Control  Voltage/1 -> Bus Creator/4, Electrical part/1(ESC voltage)  "vref"
  Bus Creator/1 -> [m5]  "m5"
  Mechanical part/1(rpm) -> RPM/1, Bus Creator/1  "rpm"
  Electrical part/1(Electrical Torque) -> Mechanical part/1(Electrical Torque)  "torque"
  Electrical part/2(current) -> ESC Current/1, Bus Creator/3  "current"
  Mechanical part/2(torque) -> Bus Creator/2  "torque"
  Mechanical part/3(angular_velocity) -> Electrical part/2(w angular speed)

== system uav_simulation_tarot_r2022a/Motors/DC Motor 6 ==
  Control  Voltage : Inport
  Bus Creator : BusCreator  Inputs=4
  Electrical part : Subsystem
  Mechanical part : Subsystem
  StaticTfric : Constant  Value=0
  RPM : Outport  VectorParamsAs1DForOutWhenUnconnected=off
  ESC Current : Outport  Port=2  VectorParamsAs1DForOutWhenUnconnected=off
  tag scope: m6=global
  wires:
  StaticTfric/1 -> Mechanical part/2(Static Friction Torque)
  Control  Voltage/1 -> Bus Creator/4, Electrical part/1(ESC voltage)  "vref"
  Bus Creator/1 -> [m6]  "m6"
  Mechanical part/1(rpm) -> RPM/1, Bus Creator/1  "rpm"
  Electrical part/1(Electrical Torque) -> Mechanical part/1(Electrical Torque)  "torque"
  Electrical part/2(current) -> ESC Current/1, Bus Creator/3  "current"
  Mechanical part/2(torque) -> Bus Creator/2  "torque"
  Mechanical part/3(angular_velocity) -> Electrical part/2(w angular speed)

== system uav_simulation_tarot_r2022a/Motors/DC Motor 7 ==
  Control  Voltage : Inport
  Bus Creator : BusCreator  Inputs=4
  Electrical part : Subsystem
  Mechanical part : Subsystem
  StaticTfric : Constant  Value=0
  RPM : Outport  VectorParamsAs1DForOutWhenUnconnected=off
  ESC Current : Outport  Port=2  VectorParamsAs1DForOutWhenUnconnected=off
  tag scope: m7=global
  wires:
  StaticTfric/1 -> Mechanical part/2(Static Friction Torque)
  Control  Voltage/1 -> Bus Creator/4, Electrical part/1(ESC voltage)  "vref"
  Bus Creator/1 -> [m7]  "m7"
  Mechanical part/1(rpm) -> RPM/1, Bus Creator/1  "rpm"
  Electrical part/1(Electrical Torque) -> Mechanical part/1(Electrical Torque)  "torque"
  Electrical part/2(current) -> ESC Current/1, Bus Creator/3  "current"
  Mechanical part/2(torque) -> Bus Creator/2  "torque"
  Mechanical part/3(angular_velocity) -> Electrical part/2(w angular speed)

== system uav_simulation_tarot_r2022a/Motors/DC Motor 8 ==
  Control  Voltage : Inport
  Bus Creator : BusCreator  Inputs=4
  Electrical part : Subsystem
  Mechanical part : Subsystem
  StaticTfric : Constant  Value=0
  RPM : Outport  VectorParamsAs1DForOutWhenUnconnected=off
  ESC Current : Outport  Port=2  VectorParamsAs1DForOutWhenUnconnected=off
  tag scope: m8=global
  wires:
  StaticTfric/1 -> Mechanical part/2(Static Friction Torque)
  Control  Voltage/1 -> Bus Creator/4, Electrical part/1(ESC voltage)  "vref"
  Bus Creator/1 -> [m8]  "m8"
  Mechanical part/1(rpm) -> RPM/1, Bus Creator/1  "rpm"
  Electrical part/1(Electrical Torque) -> Mechanical part/1(Electrical Torque)  "torque"
  Electrical part/2(current) -> ESC Current/1, Bus Creator/3  "current"
  Mechanical part/2(torque) -> Bus Creator/2  "torque"
  Mechanical part/3(angular_velocity) -> Electrical part/2(w angular speed)

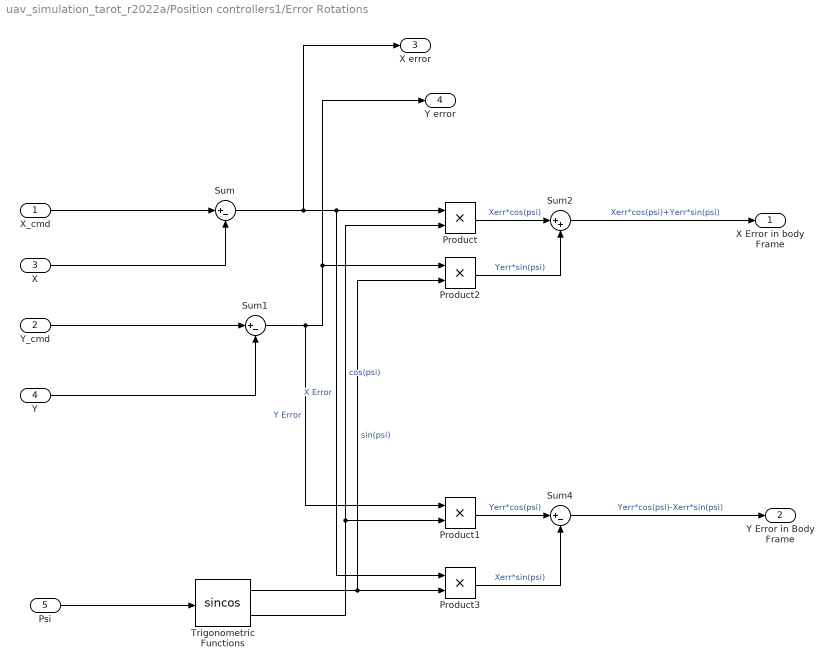
== system uav_simulation_tarot_r2022a/Position controllers1/Error Rotations ==
  X_cmd : Inport
  Y_cmd : Inport  Port=2
  X : Inport  Port=3
  Y : Inport  Port=4
  Psi : Inport  Port=5
  Product{,1..3} (4 alike) : Product
  Sum : Sum  Inputs=|+-
  Sum1 : Sum  Inputs=|+-
  Sum2 : Sum  Inputs=|++
  Sum4 : Sum  Inputs=|+-
  Trigonometric Functions : Trigonometry  Operator=sincos
  X Error in body Frame : Outport  VectorParamsAs1DForOutWhenUnconnected=off
  Y Error in Body Frame : Outport  Port=2  VectorParamsAs1DForOutWhenUnconnected=off
  X error : Outport  Port=3  VectorParamsAs1DForOutWhenUnconnected=off
  "Y error " : Outport  Port=4  VectorParamsAs1DForOutWhenUnconnected=off
  wires:
  Sum4/1 -> Y Error in Body Frame/1  "Yerr*cos(psi)-Xerr*sin(psi)"
  Product3/1 -> Sum4/2  "Xerr*sin(psi)"
  Sum1/1 -> "Y error "/1, Product2/1, Product1/1  "Y Error"
  Trigonometric Functions/1 -> Product2/2, Product3/2  "sin(psi)"
  Sum2/1 -> X Error in body Frame/1  "Xerr*cos(psi)+Yerr*sin(psi)"
  Y_cmd/1 -> Sum1/1
  X_cmd/1 -> Sum/1
  X/1 -> Sum/2
  Y/1 -> Sum1/2
  Sum/1 -> X error/1, Product3/1, Product/1  "X Error"
  Trigonometric Functions/2 -> Product/2, Product1/2  "cos(psi)"
  Product/1 -> Sum2/1  "Xerr*cos(psi)"
  Product2/1 -> Sum2/2  "Yerr*sin(psi)"
  Product1/1 -> Sum4/1  "Yerr*cos(psi)"
  Psi/1 -> Trigonometric Functions/1

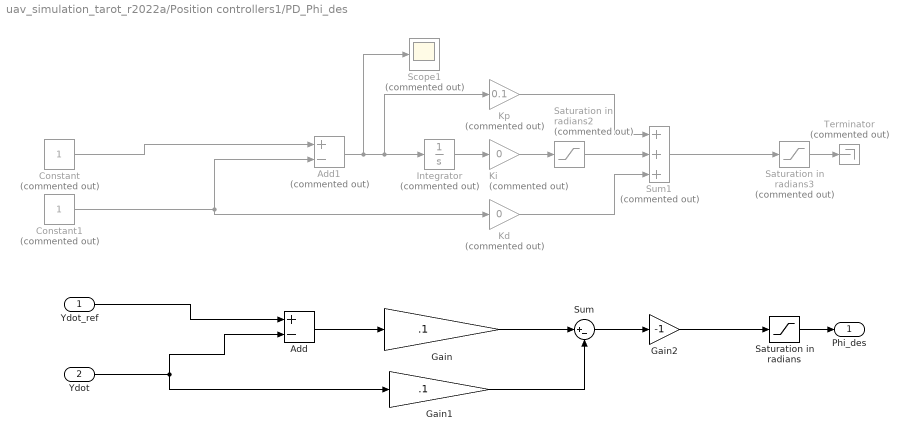
== system uav_simulation_tarot_r2022a/Position controllers1/PD_Phi_des ==
  Ydot_ref : Inport
  Ydot : Inport  Port=2
  Add : Sum  Inputs=+-
  Add1 : Sum  Commented=on  Inputs=+-
  Constant : Constant  Commented=on
  Constant1 : Constant  Commented=on
  Gain : Gain  Gain=.1
  Gain1 : Gain  Gain=.1
  Gain2 : Gain  Gain=-1
  Integrator : Integrator  Commented=on
  Kd : Gain  Commented=on  Gain=0
  Ki : Gain  Commented=on  Gain=0
  Kp : Gain  Commented=on  Gain=0.1
  Saturation in radians : Saturate  UpperLimit=40*pi/180  LowerLimit=-40*pi/180
  Saturation in radians2 : Saturate  Commented=on  UpperLimit=22*pi/180  LowerLimit=-22*pi/180
  Saturation in radians3 : Saturate  Commented=on  UpperLimit=40*pi/180  LowerLimit=-40*pi/180
  Scope1 : Scope  Commented=on
  Sum : Sum  Inputs=|+-
  Sum1 : Sum  Commented=on  Inputs=+++
  Terminator : Terminator  Commented=on
  Phi_des : Outport  VectorParamsAs1DForOutWhenUnconnected=off
  wires:
  Ydot/1 -> Add/2, Gain1/1
  Gain1/1 -> Sum/2
  Add/1 -> Gain/1
  Gain/1 -> Sum/1
  Sum/1 -> Gain2/1
  Gain2/1 -> Saturation in radians/1
  Saturation in radians3/1 -> Terminator/1
  Kd/1 -> Sum1/3
  Saturation in radians2/1 -> Sum1/2
  Integrator/1 -> Ki/1
  Constant1/1 -> Kd/1, Add1/2
  Constant/1 -> Add1/1
  Kp/1 -> Sum1/1
  Add1/1 -> Scope1/1, Integrator/1, Kp/1
  Ki/1 -> Saturation in radians2/1
  Sum1/1 -> Saturation in radians3/1
  Ydot_ref/1 -> Add/1
  Saturation in radians/1 -> Phi_des/1

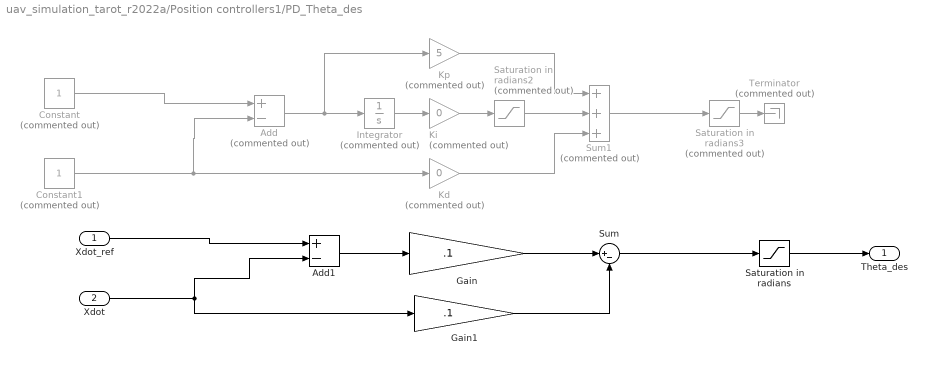
== system uav_simulation_tarot_r2022a/Position controllers1/PD_Theta_des ==
  Xdot_ref : Inport
  Xdot : Inport  Port=2
  Add : Sum  Commented=on  Inputs=+-
  Add1 : Sum  Inputs=+-
  Constant : Constant  Commented=on
  Constant1 : Constant  Commented=on
  Gain : Gain  Gain=.1
  Gain1 : Gain  Gain=.1
  Integrator : Integrator  Commented=on
  Kd : Gain  Commented=on  Gain=0
  Ki : Gain  Commented=on  Gain=0
  Kp : Gain  Commented=on  Gain=5
  Saturation in radians : Saturate  UpperLimit=40*pi/180  LowerLimit=-40*pi/180
  Saturation in radians2 : Saturate  Commented=on  UpperLimit=22*pi/180  LowerLimit=-22*pi/180
  Saturation in radians3 : Saturate  Commented=on  UpperLimit=40*pi/180  LowerLimit=-40*pi/180
  Sum : Sum  Inputs=|+-
  Sum1 : Sum  Commented=on  Inputs=+++
  Terminator : Terminator  Commented=on
  Theta_des : Outport  VectorParamsAs1DForOutWhenUnconnected=off
  wires:
  Constant/1 -> Add/1
  Saturation in radians2/1 -> Sum1/2
  Add/1 -> Integrator/1, Kp/1
  Constant1/1 -> Kd/1, Add/2
  Kp/1 -> Sum1/1
  Integrator/1 -> Ki/1
  Kd/1 -> Sum1/3
  Ki/1 -> Saturation in radians2/1
  Saturation in radians3/1 -> Terminator/1
  Sum1/1 -> Saturation in radians3/1
  Saturation in radians/1 -> Theta_des/1
  Xdot_ref/1 -> Add1/1
  Xdot/1 -> Add1/2, Gain1/1
  Gain1/1 -> Sum/2
  Sum/1 -> Saturation in radians/1
  Add1/1 -> Gain/1
  Gain/1 -> Sum/1

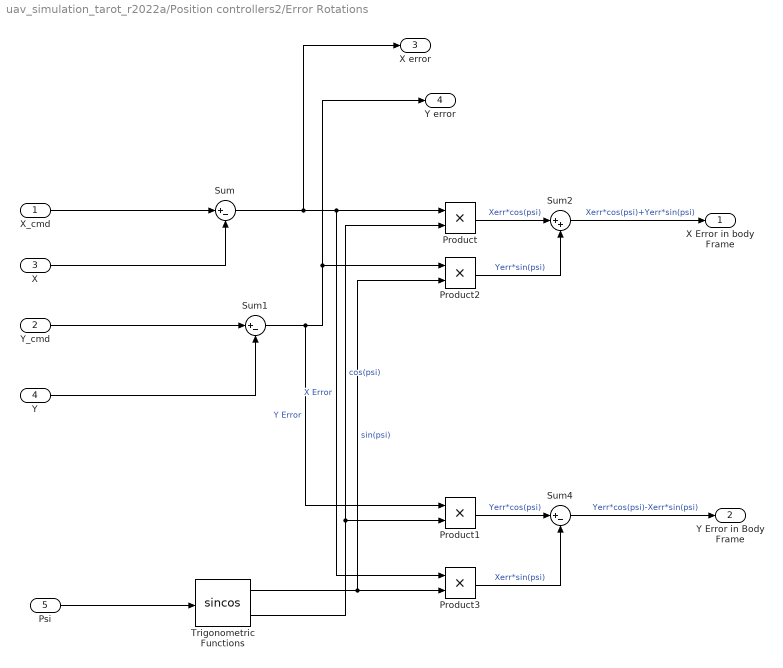
== system uav_simulation_tarot_r2022a/Position controllers2/Error Rotations ==
  X_cmd : Inport
  Y_cmd : Inport  Port=2
  X : Inport  Port=3
  Y : Inport  Port=4
  Psi : Inport  Port=5
  Product{,1..3} (4 alike) : Product
  Sum : Sum  Inputs=|+-
  Sum1 : Sum  Inputs=|+-
  Sum2 : Sum  Inputs=|++
  Sum4 : Sum  Inputs=|+-
  Trigonometric Functions : Trigonometry  Operator=sincos
  X Error in body Frame : Outport  VectorParamsAs1DForOutWhenUnconnected=off
  Y Error in Body Frame : Outport  Port=2  VectorParamsAs1DForOutWhenUnconnected=off
  X error : Outport  Port=3  VectorParamsAs1DForOutWhenUnconnected=off
  "Y error " : Outport  Port=4  VectorParamsAs1DForOutWhenUnconnected=off
  wires:
  Sum4/1 -> Y Error in Body Frame/1  "Yerr*cos(psi)-Xerr*sin(psi)"
  Product3/1 -> Sum4/2  "Xerr*sin(psi)"
  Sum1/1 -> "Y error "/1, Product2/1, Product1/1  "Y Error"
  Trigonometric Functions/1 -> Product2/2, Product3/2  "sin(psi)"
  Sum2/1 -> X Error in body Frame/1  "Xerr*cos(psi)+Yerr*sin(psi)"
  Y_cmd/1 -> Sum1/1
  X_cmd/1 -> Sum/1
  X/1 -> Sum/2
  Y/1 -> Sum1/2
  Sum/1 -> X error/1, Product3/1, Product/1  "X Error"
  Trigonometric Functions/2 -> Product/2, Product1/2  "cos(psi)"
  Product/1 -> Sum2/1  "Xerr*cos(psi)"
  Product2/1 -> Sum2/2  "Yerr*sin(psi)"
  Product1/1 -> Sum4/1  "Yerr*cos(psi)"
  Psi/1 -> Trigonometric Functions/1

== system uav_simulation_tarot_r2022a/Position controllers2/PD_Phi_des ==
  Ydot_ref : Inport
  Ydot : Inport  Port=2
  Add : Sum  Inputs=+-
  Gain : Gain  Gain=0.1
  Gain1 : Gain  Gain=0
  Gain2 : Gain  Gain=-1
  Saturation in radians : Saturate  UpperLimit=12*pi/180  LowerLimit=-12*pi/180
  Sum : Sum  Inputs=|+-
  Phi_des : Outport  VectorParamsAs1DForOutWhenUnconnected=off
  wires:
  Saturation in radians/1 -> Phi_des/1
  Ydot_ref/1 -> Add/1
  Ydot/1 -> Add/2, Gain1/1
  Gain1/1 -> Sum/2
  Add/1 -> Gain/1
  Gain/1 -> Sum/1
  Sum/1 -> Gain2/1
  Gain2/1 -> Saturation in radians/1

== system uav_simulation_tarot_r2022a/Position controllers2/PD_Theta_des ==
  Xdot_ref : Inport
  Xdot : Inport  Port=2
  Add : Sum  Inputs=+-
  Gain : Gain  Gain=0.1
  Gain1 : Gain  Gain=0
  Saturation in radians : Saturate  UpperLimit=12*pi/180  LowerLimit=-12*pi/180
  Sum : Sum  Inputs=|+-
  Theta_des : Outport  VectorParamsAs1DForOutWhenUnconnected=off
  wires:
  Sum/1 -> Saturation in radians/1
  Gain/1 -> Sum/1
  Add/1 -> Gain/1
  Gain1/1 -> Sum/2
  Xdot/1 -> Gain1/1, Add/2
  Xdot_ref/1 -> Add/1
  Saturation in radians/1 -> Theta_des/1

== system uav_simulation_tarot_r2022a/Speed Control/ESC1 ==
  Pf : Inport
  vref : Inport  Port=2
  Display{,1..3} (4 alike) : Display
  Min : MinMax  Inputs=2
  Uniform Random Number1 : UniformRandomNumber  Minimum=0  Seed=randi(100000,1)  SampleTime=10000000
  reduced output fault : MATLAB Function  TreatAsAtomicUnit=on
  y : Outport
  s : Outport  Port=2
  wires:
  vref/1 -> Min/1
  [v_batt] -> Min/2
  Min/1 -> Display/1, reduced output fault/3(u)
  Pf/1 -> Display2/1, reduced output fault/1(Pf)
  Uniform Random Number1/1 -> Display3/1, reduced output fault/2(p)
  reduced output fault/1(y) -> Display1/1, y/1
  reduced output fault/2(s) -> s/1

== system uav_simulation_tarot_r2022a/Speed Control/ESC2 ==
  Pf : Inport
  vref : Inport  Port=2
  Min : MinMax  Inputs=2
  Uniform Random Number1 : UniformRandomNumber  Minimum=0  Seed=randi(100000,1)  SampleTime=10000000
  reduced output fault : MATLAB Function  TreatAsAtomicUnit=on
  y : Outport
  s : Outport  Port=2
  wires:
  vref/1 -> Min/1
  [v_batt] -> Min/2
  Min/1 -> reduced output fault/3(u)
  Pf/1 -> reduced output fault/1(Pf)
  Uniform Random Number1/1 -> reduced output fault/2(p)
  reduced output fault/1(y) -> y/1
  reduced output fault/2(s) -> s/1

== system uav_simulation_tarot_r2022a/Speed Control/ESC3 ==
  Pf : Inport
  vref : Inport  Port=2
  Min : MinMax  Inputs=2
  Uniform Random Number1 : UniformRandomNumber  Minimum=0  Seed=randi(100000,1)  SampleTime=10000000
  reduced output fault : MATLAB Function  TreatAsAtomicUnit=on
  y : Outport
  s : Outport  Port=2
  wires:
  vref/1 -> Min/1
  [v_batt] -> Min/2
  Min/1 -> reduced output fault/3(u)
  Pf/1 -> reduced output fault/1(Pf)
  Uniform Random Number1/1 -> reduced output fault/2(p)
  reduced output fault/1(y) -> y/1
  reduced output fault/2(s) -> s/1

== system uav_simulation_tarot_r2022a/Speed Control/ESC4 ==
  Pf : Inport
  vref : Inport  Port=2
  Min : MinMax  Inputs=2
  Uniform Random Number1 : UniformRandomNumber  Minimum=0  Seed=randi(100000,1)  SampleTime=10000000
  reduced output fault : MATLAB Function  TreatAsAtomicUnit=on
  y : Outport
  s : Outport  Port=2
  wires:
  vref/1 -> Min/1
  [v_batt] -> Min/2
  Min/1 -> reduced output fault/3(u)
  Pf/1 -> reduced output fault/1(Pf)
  Uniform Random Number1/1 -> reduced output fault/2(p)
  reduced output fault/1(y) -> y/1
  reduced output fault/2(s) -> s/1

== system uav_simulation_tarot_r2022a/Speed Control/ESC5 ==
  Pf : Inport
  vref : Inport  Port=2
  Min : MinMax  Inputs=2
  Uniform Random Number1 : UniformRandomNumber  Minimum=0  Seed=randi(100000,1)  SampleTime=10000000
  reduced output fault : MATLAB Function  TreatAsAtomicUnit=on
  y : Outport
  s : Outport  Port=2
  wires:
  vref/1 -> Min/1
  [v_batt] -> Min/2
  Min/1 -> reduced output fault/3(u)
  Pf/1 -> reduced output fault/1(Pf)
  Uniform Random Number1/1 -> reduced output fault/2(p)
  reduced output fault/1(y) -> y/1
  reduced output fault/2(s) -> s/1

== system uav_simulation_tarot_r2022a/Speed Control/ESC6 ==
  Pf : Inport
  vref : Inport  Port=2
  Min : MinMax  Inputs=2
  Uniform Random Number1 : UniformRandomNumber  Minimum=0  Seed=randi(100000,1)  SampleTime=10000000
  reduced output fault : MATLAB Function  TreatAsAtomicUnit=on
  y : Outport
  s : Outport  Port=2
  wires:
  vref/1 -> Min/1
  [v_batt] -> Min/2
  Min/1 -> reduced output fault/3(u)
  Pf/1 -> reduced output fault/1(Pf)
  Uniform Random Number1/1 -> reduced output fault/2(p)
  reduced output fault/1(y) -> y/1
  reduced output fault/2(s) -> s/1

== system uav_simulation_tarot_r2022a/Speed Control/ESC7 ==
  Pf : Inport
  vref : Inport  Port=2
  Min : MinMax  Inputs=2
  Uniform Random Number1 : UniformRandomNumber  Minimum=0  Seed=randi(100000,1)  SampleTime=10000000
  reduced output fault : MATLAB Function  TreatAsAtomicUnit=on
  y : Outport
  s : Outport  Port=2
  wires:
  vref/1 -> Min/1
  [v_batt] -> Min/2
  Min/1 -> reduced output fault/3(u)
  Pf/1 -> reduced output fault/1(Pf)
  Uniform Random Number1/1 -> reduced output fault/2(p)
  reduced output fault/1(y) -> y/1
  reduced output fault/2(s) -> s/1

== system uav_simulation_tarot_r2022a/Speed Control/ESC8 ==
  Pf : Inport
  vref : Inport  Port=2
  Min : MinMax  Inputs=2
  Uniform Random Number1 : UniformRandomNumber  Minimum=0  Seed=randi(100000,1)  SampleTime=10000000
  reduced output fault : MATLAB Function  TreatAsAtomicUnit=on
  y : Outport
  s : Outport  Port=2
  wires:
  vref/1 -> Min/1
  [v_batt] -> Min/2
  Min/1 -> reduced output fault/3(u)
  Pf/1 -> reduced output fault/1(Pf)
  Uniform Random Number1/1 -> reduced output fault/2(p)
  reduced output fault/1(y) -> y/1
  reduced output fault/2(s) -> s/1

== system uav_simulation_tarot_r2022a/Motors/DC Motor 1/Electrical part ==
  ESC voltage : Inport
  w angular speed : Inport  Port=2
  1/R : Gain  Gain=1/uav.motors(1).Req
  Ke (Torque constant)1 : Gain  Gain=uav.motors(1).Ke_eq
  Kt (Torque constant) Kt=Ke for an ideal square wave motor : Gain  Gain=uav.motors(1).Ke_eq
  Saturation : Saturate  UpperLimit=uav.motors(1).current_limit  LowerLimit=0
  Sum : Sum  Inputs=|+-
  Electrical Torque : Outport  VectorParamsAs1DForOutWhenUnconnected=off
  current : Outport  Port=2  VectorParamsAs1DForOutWhenUnconnected=off
  wires:
  1/R/1 -> Saturation/1  "current i"
  Sum/1 -> 1/R/1
  Kt (Torque constant) Kt=Ke for an ideal square wave motor/1 -> Electrical Torque/1
  Ke (Torque constant)1/1 -> Sum/2
  ESC voltage/1 -> Sum/1
  w angular speed/1 -> Ke (Torque constant)1/1
  Saturation/1 -> Kt (Torque constant) Kt=Ke for an ideal square wave motor/1, current/1
